simulink library "INT_AFS_VD"  (R2016b)
settings: Solver=VariableStepAuto  StartTime=0.0  StopTime=10.0  RelTol=1e-3
settings Model: Creator=guanxiaoxing  LastModifiedBy=guanxiaoxing

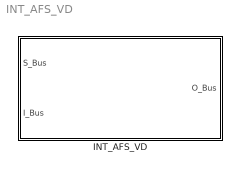
== system INT_AFS_VD ==
  INT_AFS_VD : Subsystem

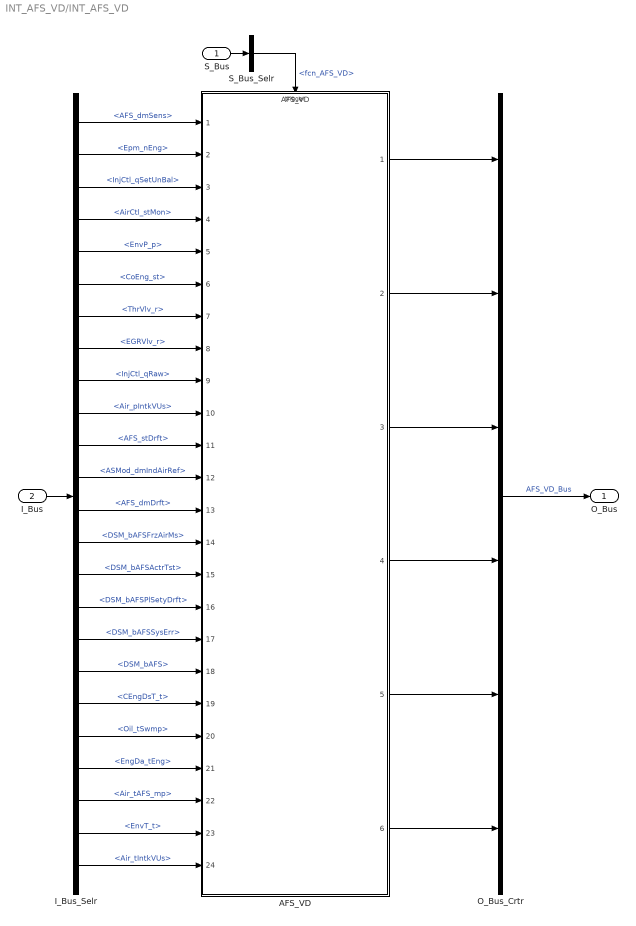
== system INT_AFS_VD/INT_AFS_VD ==
  S_Bus : Inport
  I_Bus : Inport  Port=2
  AFS_VD : ModelReference  ModelNameDialog=AFS_VD  SimulationMode=Normal  ModelReferenceVersion=1.65  TriggerPortName=function  TriggerPortTriggerType=function-call  TriggerPortStatesWhenEnabling=held
  I_Bus_Selr : BusSelector  OutputSignals=AFS_dmSens,Epm_nEng,InjCtl_qSetUnBal,AirCtl_stMon,EnvP_p,CoEng_st,ThrVlv_r,EGRVlv_r,InjCtl_qRaw,Air_pIntkVUs,AFS_stDrft,ASMod_dmIndAirRef,AFS_dmDrft,DSM_bAFSFrzAirMs,DSM_bAFSActrTst,DSM_bAFSPlSetyDrft,DSM_bAFSSysErr,DSM_bAFS,CEngDsT_t,Oil_tSwmp,EngDa_tEng,Air_tAFS_mp,EnvT_t,Air_tIntkVUs
  O_Bus_Crtr : BusCreator  Inputs=6
  S_Bus_Selr : BusSelector  OutputSignals=fcn_AFS_VD
  O_Bus : Outport
  wires:
  S_Bus_Selr/1 -> AFS_VD/Trigger  "<fcn_AFS_VD>"
  S_Bus/1 -> S_Bus_Selr/1
  I_Bus/1 -> I_Bus_Selr/1
  I_Bus_Selr/1 -> AFS_VD/1  "<AFS_dmSens>"
  I_Bus_Selr/2 -> AFS_VD/2  "<Epm_nEng>"
  I_Bus_Selr/3 -> AFS_VD/3  "<InjCtl_qSetUnBal>"
  I_Bus_Selr/4 -> AFS_VD/4  "<AirCtl_stMon>"
  I_Bus_Selr/5 -> AFS_VD/5  "<EnvP_p>"
  I_Bus_Selr/6 -> AFS_VD/6  "<CoEng_st>"
  I_Bus_Selr/7 -> AFS_VD/7  "<ThrVlv_r>"
  I_Bus_Selr/8 -> AFS_VD/8  "<EGRVlv_r>"
  I_Bus_Selr/9 -> AFS_VD/9  "<InjCtl_qRaw>"
  I_Bus_Selr/10 -> AFS_VD/10  "<Air_pIntkVUs>"
  I_Bus_Selr/11 -> AFS_VD/11  "<AFS_stDrft>"
  I_Bus_Selr/12 -> AFS_VD/12  "<ASMod_dmIndAirRef>"
  I_Bus_Selr/13 -> AFS_VD/13  "<AFS_dmDrft>"
  I_Bus_Selr/14 -> AFS_VD/14  "<DSM_bAFSFrzAirMs>"
  I_Bus_Selr/15 -> AFS_VD/15  "<DSM_bAFSActrTst>"
  I_Bus_Selr/16 -> AFS_VD/16  "<DSM_bAFSPlSetyDrft>"
  I_Bus_Selr/17 -> AFS_VD/17  "<DSM_bAFSSysErr>"
  I_Bus_Selr/18 -> AFS_VD/18  "<DSM_bAFS>"
  I_Bus_Selr/19 -> AFS_VD/19  "<CEngDsT_t>"
  I_Bus_Selr/20 -> AFS_VD/20  "<Oil_tSwmp>"
  I_Bus_Selr/21 -> AFS_VD/21  "<EngDa_tEng>"
  I_Bus_Selr/22 -> AFS_VD/22  "<Air_tAFS_mp>"
  I_Bus_Selr/23 -> AFS_VD/23  "<EnvT_t>"
  I_Bus_Selr/24 -> AFS_VD/24  "<Air_tIntkVUs>"
  O_Bus_Crtr/1 -> O_Bus/1  "AFS_VD_Bus"
  AFS_VD/1 -> O_Bus_Crtr/1
  AFS_VD/2 -> O_Bus_Crtr/2
  AFS_VD/3 -> O_Bus_Crtr/3
  AFS_VD/4 -> O_Bus_Crtr/4
  AFS_VD/5 -> O_Bus_Crtr/5
  AFS_VD/6 -> O_Bus_Crtr/6
